simulink library "BPN_lib"  (Simulink 7.4)
settings: Solver=ode45  StartTime=0.0  StopTime=10.0  RelTol=1e-3
values from neighbouring files (symbols this model uses):
  BPNc_fac_ChaPowCurLim = mpt.Parameter    [BPN_CAL.m]
  BPNc_fac_DchPowCurLim = mpt.Parameter    [BPN_CAL.m]
  BPNc_i2_ContiChaCurLim_Max = mpt.Parameter    [BPN_CAL.m]
  BPNc_i2_ContiDchCurLim_Max = mpt.Parameter    [BPN_CAL.m]
  BPNc_i_ContiChaCurLim_Max = mpt.Parameter    [BPN_CAL.m]
  BPNc_i_ContiDchCurLim_Max = mpt.Parameter    [BPN_CAL.m]
  BPNc_i_NorChaCurLim_Max = mpt.Parameter    [BPN_CAL.m]
  BPNc_i_NorDchCurLim_Max = mpt.Parameter    [BPN_CAL.m]
  BPNc_i_PackCurMeasAlwd = mpt.Parameter    [BPN_CAL.m]
  BPNc_i_SafeChaCurLim_Max = mpt.Parameter    [BPN_CAL.m]
  BPNc_i_SafeDchCurLim_Max = mpt.Parameter    [BPN_CAL.m]
  BPNc_pct_CurLimFac_warn = mpt.Parameter    [BPN_CAL.m]
  BPNc_pct_PackSocOver_fatal = mpt.Parameter    [BPN_CAL.m]
  BPNc_pct_PackSocOver_fault = mpt.Parameter    [BPN_CAL.m]
  BPNc_pct_PackSocOver_warn = mpt.Parameter    [BPN_CAL.m]
  BPNc_pct_PackSocUnder_fatal = mpt.Parameter    [BPN_CAL.m]
  BPNc_pct_PackSocUnder_fault = mpt.Parameter    [BPN_CAL.m]
  BPNc_pct_PackSocUnder_warn = mpt.Parameter    [BPN_CAL.m]
  BPNc_pct_PowLimfac_fatal = mpt.Parameter    [BPN_CAL.m]
  BPNc_pct_PowLimfac_warn = mpt.Parameter    [BPN_CAL.m]
  BPNc_r_CtrRes_fault = mpt.Parameter    [BPN_CAL.m]
  BPNc_r_PackInResThrld = mpt.Parameter    [BPN_CAL.m]
  BPNc_t_PackTemp_Mean = mpt.Parameter    [BPN_CAL.m]
  BPNc_v_CellVoltDif_fault = mpt.Parameter    [BPN_CAL.m]
  BPNc_v_CellVoltDif_warn = mpt.Parameter    [BPN_CAL.m]
  BPNc_v_CellVoltOver_fatal = mpt.Parameter    [BPN_CAL.m]
  BPNc_v_CellVoltOver_fault = mpt.Parameter    [BPN_CAL.m]
  BPNc_v_CellVoltOver_warn = mpt.Parameter    [BPN_CAL.m]
  BPNc_v_CellVoltUnder_fatal = mpt.Parameter    [BPN_CAL.m]
  BPNc_v_CellVoltUnder_fault = mpt.Parameter    [BPN_CAL.m]
  BPNc_v_CellVoltUnder_warn = mpt.Parameter    [BPN_CAL.m]
  BPNc_v_LowOPerVolt = mpt.Parameter    [BPN_CAL.m]
  BPNc_v_PackVoltDrop_fatal = mpt.Parameter    [BPN_CAL.m]
  BPNc_v_PackVoltOver_fatal = mpt.Parameter    [BPN_CAL.m]
  BPNc_v_PackVoltOver_fault = mpt.Parameter    [BPN_CAL.m]
  BPNc_v_PackVoltOver_warn = mpt.Parameter    [BPN_CAL.m]
  BPNc_v_PackVoltUnder_fatal = mpt.Parameter    [BPN_CAL.m]
  BPNc_v_PackVoltUnder_fault = mpt.Parameter    [BPN_CAL.m]
  BPNc_v_PackVoltUnder_warn = mpt.Parameter    [BPN_CAL.m]
  BPNc_v_VoltDifThrld = mpt.Parameter    [BPN_CAL.m]
  BPNy_DiagAcvnCtlCtrSt = mpt.Parameter    [BPN_CAL.m]
  BPNz_DiagAcvnCtlId = mpt.Parameter    [BPN_CAL.m]
  BSCx_BCU_State = mpt.Parameter    [BPN_CAL.m]
undefined symbols (not defined in the file or in its folder): BMS_Const_TickTm_s, BPNm_mode_DiaCtlAcv, PACK_Const_CellNumOfMdl, PACK_Const_MdlNumOfPack
libraries: Defined_Functionality x12, simulink x4
(part 1 of 2)
settings Model: Creator=lixuying  LastModifiedBy=sunsijun

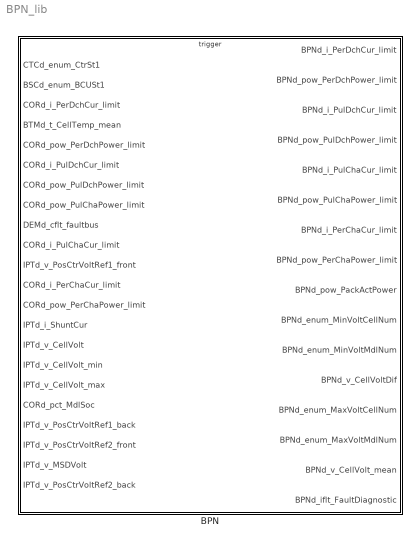
== system BPN_lib ==
  BPN : Subsystem  TreatAsAtomicUnit=on

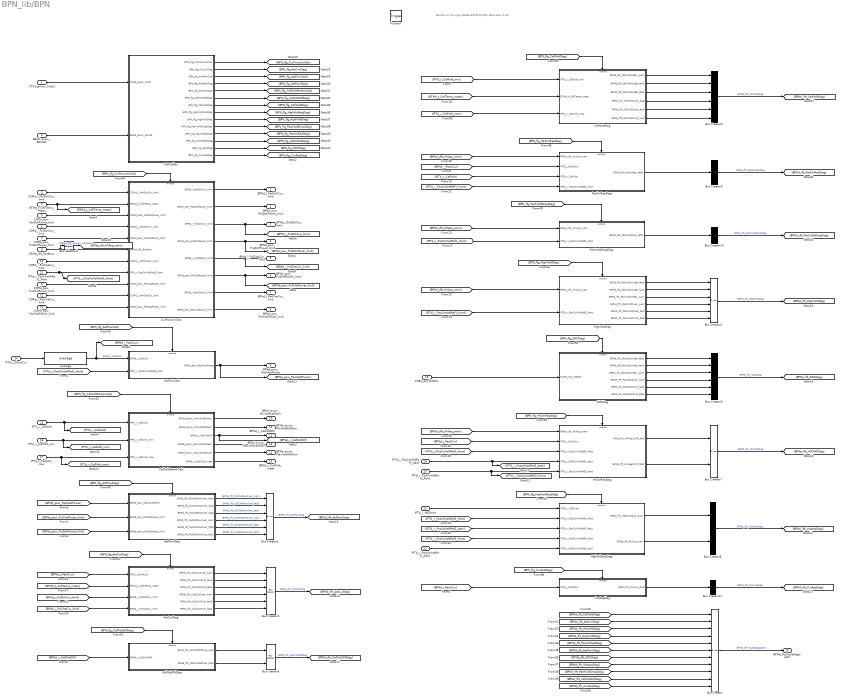
== system BPN_lib/BPN ==
  note: $Author:Li Xuying$
      | $Date:2015/11/03$
      | $Revision:1.0$
  CTCd_enum_CtrSt1 : Inport
  BSCd_enum_BCUSt1 : Inport  Port=2
  CORd_i_PerDchCur_limit : Inport  Port=3
  BTMd_t_CellTemp_mean : Inport  Port=4
  CORd_pow_PerDchPower_limit : Inport  Port=5
  CORd_i_PulDchCur_limit : Inport  Port=6
  CORd_pow_PulDchPower_limit : Inport  Port=7
  CORd_pow_PulChaPower_limit : Inport  Port=8
  DEMd_cflt_faultbus : Inport  Port=9
  CORd_i_PulChaCur_limit : Inport  Port=10
  IPTd_v_PosCtrVoltRef1_front : Inport  Port=11
  CORd_i_PerChaCur_limit : Inport  Port=12
  CORd_pow_PerChaPower_limit : Inport  Port=13
  IPTd_i_ShuntCur : Inport  Port=14
  IPTd_v_CellVolt : Inport  Port=15
  IPTd_v_CellVolt_min : Inport  Port=16
  IPTd_v_CellVolt_max : Inport  Port=17
  CORd_pct_MdlSoc : Inport  Port=18
  IPTd_v_PosCtrVoltRef1_back : Inport  Port=19
  IPTd_v_PosCtrVoltRef2_front : Inport  Port=20
  IPTd_v_MSDVolt : Inport  Port=21
  IPTd_v_PosCtrVoltRef2_back : Inport  Port=22
  function : TriggerPort  TriggerType=function-call
  ActCurDiag : Subsystem
  ActPowCalc : Subsystem
  ActPowDiag : Subsystem
  Bus Creator : BusCreator  Inputs=11
  Bus Creator{1..5} (5 alike) : BusCreator  Inputs=6
  Bus Creator10 : BusCreator  Inputs=1
  Bus Creator11 : BusCreator  Inputs=1
  Bus Creator6 : BusCreator  Inputs=2
  Bus Creator7 : BusCreator  Inputs=2
  Bus Creator8 : BusCreator  Inputs=2
  Bus Creator9 : BusCreator  Inputs=1
  Bus Selector3 : BusSelector  OutputSignals=BPN_Fault_Bus.BPNd_cflt_HVAcq_warnRaw
  CellVoltDiag : Subsystem
  CellVoltDifDiag : Subsystem
  CellVoltParamCalc : Subsystem
  CurAcqDiag : Subsystem
  CurPowLimCalc : Subsystem
  DiaCtrlAcv : Subsystem  TreatAsAtomicUnit=on
  HVCtrResDiag : Subsystem
  HighVoltAcqDiag : Subsystem
  HighVoltDiag : Subsystem
  PackInResDiag : Subsystem
  PackVoltDropDiag : Subsystem
  SOCDiag : Subsystem
  average : Defined_Functionality/average  SystemSampleTime=-1  time=50  period=10
      settings: AttributesFormatString=[TIME_ms=%<time>]\n[PERIOD_ms=%<period>]
  BPNd_i_PerDchCur_limit : Outport
  BPNd_pow_PerDchPower_limit : Outport  Port=2
  BPNd_i_PulDchCur_limit : Outport  Port=3
  BPNd_pow_PulDchPower_limit : Outport  Port=4
  BPNd_i_PulChaCur_limit : Outport  Port=5
  BPNd_pow_PulChaPower_limit : Outport  Port=6
  BPNd_i_PerChaCur_limit : Outport  Port=7
  BPNd_pow_PerChaPower_limit : Outport  Port=8
  BPNd_pow_PackActPower : Outport  Port=9
  BPNd_enum_MinVoltCellNum : Outport  Port=10
  BPNd_enum_MinVoltMdlNum : Outport  Port=11
  BPNd_v_CellVoltDif : Outport  Port=12
  BPNd_enum_MaxVoltCellNum : Outport  Port=13
  BPNd_enum_MaxVoltMdlNum : Outport  Port=14
  BPNd_v_CellVolt_mean : Outport  Port=15
  BPNd_iflt_FaultDiagnostic : Outport  Port=16
  wires:
  CellVoltDiag/6(BPNd_iflt_CellVoltOver_warn) -> Bus Creator3/6
  CellVoltDiag/4(BPNd_iflt_CellVoltOver_fatal) -> Bus Creator3/4
  CurPowLimCalc/6(BPNd_pow_PulChaPower_limit) -> [BPNd_pow_PulChaPower_limit], BPNd_pow_PulChaPower_limit/1
  CurPowLimCalc/5(BPNd_i_PulChaCur_limit) -> [BPNd_i_PulChaCur_limit], BPNd_i_PulChaCur_limit/1
  CurPowLimCalc/4(BPNd_pow_PulDchPower_limit) -> [BPNd_pow_PulDchPower_limit], BPNd_pow_PulDchPower_limit/1
  CurPowLimCalc/3(BPNd_i_PulDchCur_limit) -> [BPNd_i_PulDchCur_limit], BPNd_i_PulDchCur_limit/1
  CurPowLimCalc/2(BPNd_pow_PerDchPower_limit) -> BPNd_pow_PerDchPower_limit/1
  CurPowLimCalc/1(BPNd_i_PerDchCur_limit) -> BPNd_i_PerDchCur_limit/1
  [BPN_flg_HVCtrResDiag] -> HVCtrResDiag/Enable
  [BPN_flg_HighVoltAcqDiag] -> HighVoltAcqDiag/Enable
  DiaCtrlAcv/14(BPN_flg_CurAcqDiag) -> [BPN_flg_CurAcqDiag]
  DiaCtrlAcv/13(BPN_flg_SOCDiag) -> [BPN_flg_SOCDiag]
  DiaCtrlAcv/12(BPN_flg_HVCtrResDiag) -> [BPN_flg_HVCtrResDiag]
  DiaCtrlAcv/11(BPN_flg_PackInResDiag) -> [BPN_flg_PackInResDiag]
  DiaCtrlAcv/10(BPN_flg_PackVoltDropDiag) -> [BPN_flg_PackVoltDropDiag]
  DiaCtrlAcv/9(BPN_flg_HighVoltDiag) -> [BPN_flg_HighVoltDiag]
  DiaCtrlAcv/8(BPN_flg_HighVoltAcqDiag) -> [BPN_flg_HighVoltAcqDiag]
  DiaCtrlAcv/7(BPN_flg_CellVoltDiag) -> [BPN_flg_CellVoltDiag]
  DiaCtrlAcv/6(BPN_flg_CellVoltDifDiag) -> [BPN_flg_CellVoltDifDiag]
  DiaCtrlAcv/5(BPN_flg_CellVoltCalc) -> [BPN_flg_CellVoltParamCalc]
  DiaCtrlAcv/4(BPN_flg_ActPowDiag) -> [BPN_flg_ActPowDiag]
  DiaCtrlAcv/3(BPN_flg_ActPowCalc) -> [BPN_flg_ActPowCalc]
  DiaCtrlAcv/2(BPN_flg_ActCurDiag) -> [BPN_flg_ActCurDiag]
  DiaCtrlAcv/1(BPN_flg_CurPowLimCalc) -> [BPN_flg_CurPowLimCalc]
  Bus Selector3/1 -> [BPNd_cflt_HVAcq_warn]  "<BPNd_cflt_HVAcq_warnRaw>"
  [IPTd_v_PosCtrVoltRef1_back] -> HighVoltAcqDiag/3(IPTd_v_PosCtrVoltRef1_back)
  [IPTd_v_PosCtrVoltRef1_front] -> HighVoltAcqDiag/2(IPTd_v_PosCtrVoltRef1_front)
  IPTd_v_PosCtrVoltRef2_back/1 -> HighVoltAcqDiag/5(IPTd_v_PosCtrVoltRef2_back)
  [IPTd_v_PosCtrVoltRef2_front] -> HighVoltAcqDiag/4(IPTd_v_PosCtrVoltRef2_front)
  HighVoltAcqDiag/1(BPNd_iflt_MSDVoltAcq_warn) -> Bus Creator8/1
  HighVoltAcqDiag/2(BPNd_iflt_HVAcq_warn) -> Bus Creator8/2
  [BPN_flg_CellVoltParamCalc] -> CellVoltParamCalc/Enable
  [BPN_flg_SOCDiag] -> SOCDiag/Enable
  CTCd_enum_CtrSt1/1 -> DiaCtrlAcv/1(CTCd_enum_CtrSt)
  BSCd_enum_BCUSt1/1 -> DiaCtrlAcv/2(BSCd_enum_BCUSt)
  ActPowCalc/1(BPNd_pow_PackActPower) -> [BPNd_pow_PackActPower], BPNd_pow_PackActPower/1
  SOCDiag/6(BPNd_iflt_PackSocOver_fatal) -> Bus Creator5/6
  SOCDiag/5(BPNd_iflt_PackSocOver_fault) -> Bus Creator5/5
  SOCDiag/4(BPNd_iflt_PackSocOver_warn) -> Bus Creator5/4
  SOCDiag/3(BPNd_iflt_PackSocUnder_warn) -> Bus Creator5/3
  SOCDiag/2(BPNd_iflt_PackSocUnder_fault) -> Bus Creator5/2
  SOCDiag/1(BPNd_iflt_PackSocUnder_fatal) -> Bus Creator5/1
  HighVoltDiag/6(BPNd_iflt_PackVoltOver_fatal) -> Bus Creator4/6
  HighVoltDiag/5(BPNd_iflt_PackVoltOver_fault) -> Bus Creator4/5
  HighVoltDiag/4(BPNd_iflt_PackVoltOver_warn) -> Bus Creator4/4
  HighVoltDiag/3(BPNd_iflt_PackVoltUnder_warn) -> Bus Creator4/3
  HighVoltDiag/2(BPNd_iflt_PackVoltUnder_fault) -> Bus Creator4/2
  HighVoltDiag/1(BPNd_iflt_PackVoltUnder_fatal) -> Bus Creator4/1
  CellVoltParamCalc/3(BPNd_v_CellVoltDif) -> [BPNd_v_CellVoltDif], BPNd_v_CellVoltDif/1
  BTMd_t_CellTemp_mean/1 -> [BTMd_t_CellTemp_mean], CurPowLimCalc/2(BTMd_t_CellTemp_mean)
  CORd_pow_PulDchPower_limit/1 -> CurPowLimCalc/5(CORd_pow_PulDchPower_limit)
  CORd_pow_PerDchPower_limit/1 -> CurPowLimCalc/3(CORd_pow_PerDchPower_limit)
  CORd_i_PulChaCur_limit/1 -> CurPowLimCalc/7(CORd_i_PulChaCur_limit)
  CORd_i_PerChaCur_limit/1 -> CurPowLimCalc/10(CORd_i_PerChaCur_limit)
  CORd_pow_PerChaPower_limit/1 -> CurPowLimCalc/11(CORd_pow_PerChaPower_limit)
  CORd_pow_PulChaPower_limit/1 -> CurPowLimCalc/9(CORd_pow_PulChaPower_limit)
  CORd_i_PulDchCur_limit/1 -> CurPowLimCalc/4(CORd_i_PulDchCur_limit)
  CORd_i_PerDchCur_limit/1 -> CurPowLimCalc/1(CORd_i_PerDchCur_limit)
  IPTd_v_PosCtrVoltRef2_front/1 -> [IPTd_v_PosCtrVoltRef2_front], HVCtrResDiag/5(IPTd_v_PosCtrVoltRef2_front)
  IPTd_v_PosCtrVoltRef1_back/1 -> [IPTd_v_PosCtrVoltRef1_back], HVCtrResDiag/4(IPTd_v_PosCtrVoltRef1_back)
  [BPNd_i_PackCur] -> CurAcqDiag/1(IPTd_i_ShuntCur)
  average/1 -> [BPNd_i_PackCur], ActPowCalc/1(BPNd_i_PackCur)  "BPNd_i_PackCur"
  IPTd_v_CellVolt_max/1 -> [IPTd_v_CellVolt_max], CellVoltParamCalc/3(IPTd_v_CellVolt_max)
  [IPTd_v_CellVolt_max] -> CellVoltDiag/3(IPTd_v_CellVolt_max)
  [IPTd_v_CellVolt_min] -> CellVoltDiag/1(IPTd_v_CellVolt_min)
  IPTd_v_CellVolt_min/1 -> [IPTd_v_CellVolt_min], CellVoltParamCalc/2(IPTd_v_CellVolt_min)
  [BPNd_iflt_CurAcqDiag] -> Bus Creator/11
  Bus Creator11/1 -> [BPNd_iflt_CurAcqDiag]  "BPNd_iflt_CurAcqDiag"
  [BPN_flg_CurAcqDiag] -> CurAcqDiag/Enable
  CurAcqDiag/1(BPNd_iflt_CurAcq_fault) -> Bus Creator11/1
  HVCtrResDiag/2(BPNd_iflt_HVNegCtrlR_fault) -> Bus Creator7/2
  HVCtrResDiag/1(BPNd_iflt_HVPosCtrlR_fault) -> Bus Creator7/1
  IPTd_v_MSDVolt/1 -> HighVoltAcqDiag/1(IPTd_v_MSDVolt)
  [BPNd_cflt_HVAcq_warn] -> PackVoltDropDiag/1(BPNd_cflt_HVAcq_warn)
  [IPTd_v_PosCtrVoltRef1_front] -> PackVoltDropDiag/2(IPTd_v_PosCtrVoltRef1_front)
  [IPTd_v_PosCtrVoltRef1_front] -> HighVoltDiag/2(IPTd_v_PosCtrVoltRef1_front)
  DEMd_cflt_faultbus/1 -> Bus Selector3/1, CurPowLimCalc/6(DEMd_cflt_faultbus)
  CurPowLimCalc/8(BPNd_pow_PerChaPower_limit) -> BPNd_pow_PerChaPower_limit/1
  IPTd_i_ShuntCur/1 -> average/1
  [IPTd_v_PosCtrVoltRef1_front] -> ActPowCalc/2(IPTd_v_PosCtrVoltRef1_front)
  [BPNd_pow_PulChaPower_limit] -> ActPowDiag/2(BPNd_pow_PulChaPower_limit)
  [BPNd_pow_PulDchPower_limit] -> ActPowDiag/3(BPNd_pow_PulDchPower_limit)
  [BPNd_pow_PackActPower] -> ActPowDiag/1(BPNd_pow_PackActPower)
  CORd_pct_MdlSoc/1 -> SOCDiag/1(CORd_pct_MdlSoc)
  CellVoltParamCalc/6(BPNd_v_CellVolt_mean) -> BPNd_v_CellVolt_mean/1
  CellVoltParamCalc/1(BPNd_enum_MinVoltCellNum) -> BPNd_enum_MinVoltCellNum/1
  CellVoltParamCalc/2(BPNd_enum_MinVoltMdlNum) -> BPNd_enum_MinVoltMdlNum/1
  CellVoltParamCalc/4(BPNd_enum_MaxVoltCellNum) -> BPNd_enum_MaxVoltCellNum/1
  CellVoltParamCalc/5(BPNd_enum_MaxVoltMdlNum) -> BPNd_enum_MaxVoltMdlNum/1
  [BPNd_v_CellVoltDif] -> CellVoltDifDiag/1(BPNd_v_CellVoltDif)
  CellVoltDifDiag/1(BPNd_iflt_CellVoltDifOver_warn) -> Bus Creator6/1
  CellVoltDifDiag/2(BPNd_iflt_CellVoltDifOver_fault) -> Bus Creator6/2
  [BPNd_i_PackCur] -> ActCurDiag/1(IPTd_i_ShuntCur)
  IPTd_v_CellVolt/1 -> [IPTd_v_CellVolt], CellVoltParamCalc/1(IPTd_v_CellVolt)
  PackInResDiag/1(BPNd_iflt_PackInRes_fatal) -> Bus Creator9/1
  [BPNd_i_PackCur] -> PackInResDiag/2(IPTd_i_ShuntCur)
  [IPTd_v_CellVolt] -> PackInResDiag/3(IPTd_v_CellVolt)
  IPTd_v_PosCtrVoltRef1_front/1 -> CurPowLimCalc/8(IPTd_v_PosCtrVoltRef1_front), [IPTd_v_PosCtrVoltRef1_front]
  [IPTd_v_PosCtrVoltRef1_front] -> PackInResDiag/4(IPTd_v_PosCtrVoltRef1_front)
  [BPNd_i_PackCur] -> HVCtrResDiag/2(IPTd_i_ShuntCur)
  [IPTd_v_PosCtrVoltRef1_front] -> HVCtrResDiag/3(IPTd_v_PosCtrVoltRef1_front)
  [BTMd_t_CellTemp_mean] -> ActCurDiag/2(BTMd_t_CellTemp_mean)
  [BTMd_t_CellTemp_mean] -> CellVoltDiag/2(BTMd_t_CellTemp_mean)
  [BPNd_i_PulDchCur_limit] -> ActCurDiag/3(BPNd_i_PulDchCur_limit)
  [BPNd_i_PulChaCur_limit] -> ActCurDiag/4(BPNd_i_PulChaCur_limit)
  CurPowLimCalc/7(BPNd_i_PerChaCur_limit) -> BPNd_i_PerChaCur_limit/1
  ActPowDiag/1(BPNd_iflt_PulChaPowOver_warn) -> Bus Creator1/1  "BPNd_iflt_PulChaPowOver_warn"
  ActPowDiag/2(BPNd_iflt_PulChaPowOver_fault) -> Bus Creator1/2  "BPNd_iflt_PulChaPowOver_fault"
  ActPowDiag/3(BPNd_iflt_PulChaPowOver_fatal) -> Bus Creator1/3  "BPNd_iflt_PulChaPowOver_fatal"
  ActPowDiag/4(BPNd_iflt_PulDchPowOver_warn) -> Bus Creator1/4  "BPNd_iflt_PulDchPowOver_warn"
  ActPowDiag/5(BPNd_iflt_PulDchPowOver_fatal) -> Bus Creator1/5  "BPNd_iflt_PulDchPowOver_fatal"
  ActPowDiag/6(BPNd_iflt_PulDchPowOver_fault) -> Bus Creator1/6  "BPNd_iflt_PulDchPowOver_fault"
  [BPNd_cflt_HVAcq_warn] -> HVCtrResDiag/1(BPNd_cflt_HVAcq_warn)
  PackVoltDropDiag/1(BPNd_ilft_PackVoltDrop_fatal) -> Bus Creator10/1
  [BPNd_cflt_HVAcq_warn] -> PackInResDiag/1(BPNd_cflt_HVAcq_warn)
  [BPNd_cflt_HVAcq_warn] -> HighVoltDiag/1(BPNd_cflt_HVAcq_warn)
  Bus Creator/1 -> BPNd_iflt_FaultDiagnostic/1  "BPNd_iflt_FaultDiagnostic"
  Bus Creator1/1 -> [BPNd_iflt_ActPowDiag]  "BPNd_iflt_ActPowDiag"
  ActCurDiag/1(BPNd_iflt_DchCurOver_warn) -> Bus Creator2/1
  ActCurDiag/2(BPNd_iflt_DchCurOver_fault) -> Bus Creator2/2
  ActCurDiag/3(BPNd_iflt_DchCurOver_fatal) -> Bus Creator2/3
  ActCurDiag/4(BPNd_iflt_ChaCurOver_warn) -> Bus Creator2/4
  ActCurDiag/5(BPNd_iflt_ChaCurOver_fault) -> Bus Creator2/5
  ActCurDiag/6(BPNd_iflt_ChaCurOver_fatal) -> Bus Creator2/6
  Bus Creator2/1 -> [BPNd_iflt_ActCurDiag]  "BPNd_iflt_ActCurDiag"
  Bus Creator3/1 -> [BPNd_iflt_CellVoltDiag]  "BPNd_iflt_CellVoltDiag"
  CellVoltDiag/1(BPNd_iflt_CellVoltUnder_warn) -> Bus Creator3/1
  CellVoltDiag/2(BPNd_iflt_CellVoltUnder_fault) -> Bus Creator3/2
  CellVoltDiag/3(BPNd_iflt_CellVoltUnder_fatal) -> Bus Creator3/3
  CellVoltDiag/5(BPNd_iflt_CellVoltOver_fault) -> Bus Creator3/5
  Bus Creator4/1 -> [BPNd_iflt_HighVoltDiag]  "BPNd_iflt_HighVoltDiag"
  Bus Creator5/1 -> [BPNd_iflt_SOCDiag]  "BPNd_iflt_SOCDiag"
  Bus Creator7/1 -> [BPNd_iflt_HVCtrRDiag]  "BPNd_iflt_HVCtrRDiag"
  [BPNd_iflt_CellVoltDiag] -> Bus Creator/1
  [BPNd_iflt_ActCurDiag] -> Bus Creator/2
  [BPNd_iflt_HVCtrRDiag] -> Bus Creator/3
  [BPNd_iflt_HighVoltDiag] -> Bus Creator/4
  [BPNd_iflt_PackInResDiag] -> Bus Creator/5
  [BPNd_iflt_ActPowDiag] -> Bus Creator/6
  [BPNd_iflt_SOCDiag] -> Bus Creator/7
  [BPNd_iflt_VoltAcqDiag] -> Bus Creator/8
  [BPNd_ilft_PackVoltDropDiag] -> Bus Creator/9
  Bus Creator6/1 -> [BPNd_iflt_CellVoltDifDiag]  "BPNd_iflt_CellVoltDifDiag"
  Bus Creator8/1 -> [BPNd_iflt_VoltAcqDiag]  "BPNd_iflt_VoltAcqDiag"
  Bus Creator9/1 -> [BPNd_iflt_PackInResDiag]  "BPNd_iflt_PackInResDiag"
  Bus Creator10/1 -> [BPNd_ilft_PackVoltDropDiag]  "BPNd_ilft_PackVoltDropDiag"
  [BPNd_iflt_CellVoltDifDiag] -> Bus Creator/10
  [BPN_flg_CurPowLimCalc] -> CurPowLimCalc/Enable
  [BPN_flg_ActPowCalc] -> ActPowCalc/Enable
  [BPN_flg_ActPowDiag] -> ActPowDiag/Enable
  [BPN_flg_ActCurDiag] -> ActCurDiag/Enable
  [BPN_flg_PackInResDiag] -> PackInResDiag/Enable
  [BPN_flg_PackVoltDropDiag] -> PackVoltDropDiag/Enable
  [BPN_flg_CellVoltDiag] -> CellVoltDiag/Enable
  [BPN_flg_CellVoltDifDiag] -> CellVoltDifDiag/Enable
  [BPN_flg_HighVoltDiag] -> HighVoltDiag/Enable

== system BPN_lib/BPN/ActCurDiag ==
  IPTd_i_ShuntCur : Inport
  BTMd_t_CellTemp_mean : Inport  Port=2
  BPNd_i_PulDchCur_limit : Inport  Port=3
  BPNd_i_PulChaCur_limit : Inport  Port=4
  Enable : EnablePort
  ChaCurDiag : Subsystem  TreatAsAtomicUnit=on
  DchCurDiag : Subsystem  TreatAsAtomicUnit=on
  If : If
  Subsystem : Subsystem
  BPNd_iflt_DchCurOver_warn : Outport
  BPNd_iflt_DchCurOver_fault : Outport  Port=2
  BPNd_iflt_DchCurOver_fatal : Outport  Port=3
  BPNd_iflt_ChaCurOver_warn : Outport  Port=4
  BPNd_iflt_ChaCurOver_fault : Outport  Port=5
  BPNd_iflt_ChaCurOver_fatal : Outport  Port=6
  wires:
  [BPN_i_PulChaCur_LimitAbs] -> ChaCurDiag/3(BPNd_i_PulChaCur_limit)
  [BTMd_t_CellTemp_mean] -> ChaCurDiag/1(BTMd_t_CellTemp_mean)
  Subsystem/1(BPN_i_PulDchCur_limit) -> DchCurDiag/2(BPNd_i_PulDchCur_limit)
  BTMd_t_CellTemp_mean/1 -> [BTMd_t_CellTemp_mean], DchCurDiag/3(BTMd_t_CellTemp_mean)
  BPNd_i_PulChaCur_limit/1 -> Subsystem/2(BPNd_i_PulChaCur_limit)
  Subsystem/2(BPN_i_PulChaCur_LimitAbs) -> [BPN_i_PulChaCur_LimitAbs]
  BPNd_i_PulDchCur_limit/1 -> Subsystem/1(BPNd_i_PulDchCur_limit)
  ChaCurDiag/1(BPNd_iflt_ChaCurOver_fault) -> BPNd_iflt_ChaCurOver_fault/1
  ChaCurDiag/2(BPNd_iflt_ChaCurOver_warn) -> BPNd_iflt_ChaCurOver_warn/1
  [IPTd_i_ShuntCur] -> ChaCurDiag/2(IPTd_i_ShuntCur)
  [IPTd_i_ShuntCur] -> DchCurDiag/1(IPTd_i_PackCur)
  IPTd_i_ShuntCur/1 -> [IPTd_i_ShuntCur], If/1
  ChaCurDiag/3(BPNd_iflt_ChaCurOver_fatal) -> BPNd_iflt_ChaCurOver_fatal/1
  DchCurDiag/3(BPNd_iflt_DchCurOver_fatal) -> BPNd_iflt_DchCurOver_fatal/1
  DchCurDiag/1(BPNd_iflt_DchCurOver_warn) -> BPNd_iflt_DchCurOver_warn/1
  DchCurDiag/2(BPNd_iflt_DchCurOver_fault) -> BPNd_iflt_DchCurOver_fault/1
  If/2 -> ChaCurDiag/Action
  If/1 -> DchCurDiag/Action

== system BPN_lib/BPN/ActPowCalc ==
  BPNd_i_PackCur : Inport
  IPTd_v_PosCtrVoltRef1_front : Inport  Port=2
  Enable : EnablePort
  Product : Product  RndMeth=Zero
  BPNd_pow_PackActPower : Outport
  wires:
  IPTd_v_PosCtrVoltRef1_front/1 -> Product/2
  Product/1 -> BPNd_pow_PackActPower/1  "BPNd_pow_PackActPower"
  BPNd_i_PackCur/1 -> Product/1

== system BPN_lib/BPN/ActPowDiag ==
  BPNd_pow_PackActPower : Inport
  BPNd_pow_PulChaPower_limit : Inport  Port=2
  BPNd_pow_PulDchPower_limit : Inport  Port=3
  Enable : EnablePort
  If : If  IfExpression=u1 < 0
  PulChaPower_Diagnosic : Subsystem  TreatAsAtomicUnit=on
  PulDchPower_Diagnosic : Subsystem  TreatAsAtomicUnit=on
  BPNd_iflt_PulChaPowOver_warn : Outport  DataType=boolean  OutDataTypeStr=boolean
  BPNd_iflt_PulChaPowOver_fault : Outport  Port=2  DataType=boolean  OutDataTypeStr=boolean
  BPNd_iflt_PulChaPowOver_fatal : Outport  Port=3  DataType=boolean  OutDataTypeStr=boolean
  BPNd_iflt_PulDchPowOver_warn : Outport  Port=4  DataType=boolean  OutDataTypeStr=boolean
  BPNd_iflt_PulDchPowOver_fatal : Outport  Port=5  DataType=boolean  OutDataTypeStr=boolean
  BPNd_iflt_PulDchPowOver_fault : Outport  Port=6  DataType=boolean  OutDataTypeStr=boolean  InitialOutput=0
  wires:
  [BPNd_pow_PackActPower] -> PulDchPower_Diagnosic/2(BPNd_pow_PackActPower)
  [BPNd_pow_PackActPower] -> PulChaPower_Diagnosic/1(BPNd_pow_PackActPower)
  BPNd_pow_PulChaPower_limit/1 -> PulChaPower_Diagnosic/2(BPNd_pow_PulChaPower_limit)
  PulChaPower_Diagnosic/3(BPNd_iflt_PulChaPowOver_fatal) -> BPNd_iflt_PulChaPowOver_fatal/1
  PulChaPower_Diagnosic/2(BPNd_iflt_PulChaPowOver_fault) -> BPNd_iflt_PulChaPowOver_fault/1
  PulChaPower_Diagnosic/1(BPNd_iflt_PulChaPowOver_warn) -> BPNd_iflt_PulChaPowOver_warn/1
  PulDchPower_Diagnosic/2(BPNd_iflt_PulDchPowOver_fault) -> BPNd_iflt_PulDchPowOver_fault/1
  BPNd_pow_PackActPower/1 -> [BPNd_pow_PackActPower], If/1
  PulDchPower_Diagnosic/1(BPNd_iflt_PulDchPowOver_warn) -> BPNd_iflt_PulDchPowOver_warn/1
  PulDchPower_Diagnosic/3(BPNd_iflt_PulDchPowOver_fatal) -> BPNd_iflt_PulDchPowOver_fatal/1
  BPNd_pow_PulDchPower_limit/1 -> PulDchPower_Diagnosic/1(BPNd_pow_PulDchPower_limit)
  If/1 -> PulChaPower_Diagnosic/Action
  If/2 -> PulDchPower_Diagnosic/Action

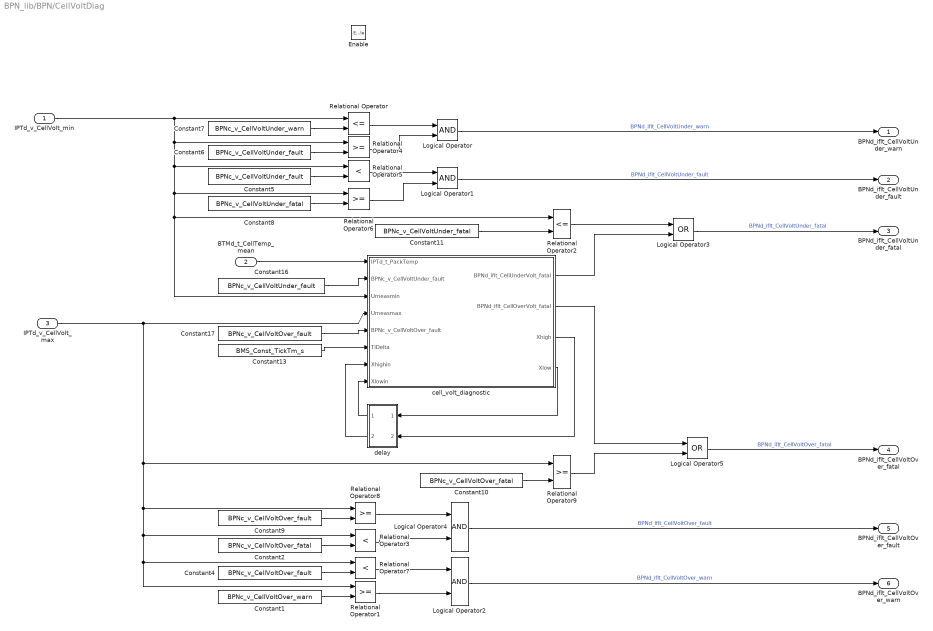
== system BPN_lib/BPN/CellVoltDiag ==
  IPTd_v_CellVolt_min : Inport
  BTMd_t_CellTemp_mean : Inport  Port=2
  IPTd_v_CellVolt_max : Inport  Port=3
  Enable : EnablePort
  Constant1 : Constant  Value=BPNc_v_CellVoltOver_warn
  Constant10 : Constant  Value=BPNc_v_CellVoltOver_fatal
  Constant11 : Constant  Value=BPNc_v_CellVoltUnder_fatal
  Constant13 : Constant  Value=BMS_Const_TickTm_s  OutDataTypeMode=single  OutDataTypeStr=single
  Constant16 : Constant  Value=BPNc_v_CellVoltUnder_fault  OutDataTypeMode=single  OutDataTypeStr=single
  Constant17 : Constant  Value=BPNc_v_CellVoltOver_fault  OutDataTypeMode=single  OutDataTypeStr=single
  Constant2 : Constant  Value=BPNc_v_CellVoltOver_fatal
  Constant4 : Constant  Value=BPNc_v_CellVoltOver_fault
  Constant5 : Constant  Value=BPNc_v_CellVoltUnder_fault
  Constant6 : Constant  Value=BPNc_v_CellVoltUnder_fault
  Constant7 : Constant  Value=BPNc_v_CellVoltUnder_warn
  Constant8 : Constant  Value=BPNc_v_CellVoltUnder_fatal
  Constant9 : Constant  Value=BPNc_v_CellVoltOver_fault
  Logical Operator{,1..2,4} (4 alike) : Logic  AllPortsSameDT=off  OutDataTypeMode=boolean  OutDataTypeStr=boolean
  Logical Operator3 : Logic  Operator=OR  AllPortsSameDT=off  OutDataTypeMode=boolean  OutDataTypeStr=boolean
  Logical Operator5 : Logic  Operator=OR  AllPortsSameDT=off  OutDataTypeMode=boolean  OutDataTypeStr=boolean
  Relational Operator : RelationalOperator  Operator=<=  LogicOutDataTypeMode=boolean  OutDataTypeStr=boolean
  Relational Operator{1,4,6,8..9} (5 alike) : RelationalOperator  LogicOutDataTypeMode=boolean  OutDataTypeStr=boolean
  Relational Operator2 : RelationalOperator  Operator=<=  LogicOutDataTypeMode=boolean  OutDataTypeStr=boolean
  Relational Operator3 : RelationalOperator  Operator=<  LogicOutDataTypeMode=boolean  OutDataTypeStr=boolean
  Relational Operator5 : RelationalOperator  Operator=<  LogicOutDataTypeMode=boolean  OutDataTypeStr=boolean
  Relational Operator7 : RelationalOperator  Operator=<  LogicOutDataTypeMode=boolean  OutDataTypeStr=boolean
  cell_volt_diagnostic : Stateflow chart  TreatAsAtomicUnit=on
  delay : Subsystem
  BPNd_iflt_CellVoltUnder_warn : Outport
  BPNd_iflt_CellVoltUnder_fault : Outport  Port=2
  BPNd_iflt_CellVoltUnder_fatal : Outport  Port=3
  BPNd_iflt_CellVoltOver_fatal : Outport  Port=4
  BPNd_iflt_CellVoltOver_fault : Outport  Port=5
  BPNd_iflt_CellVoltOver_warn : Outport  Port=6
  wires:
  IPTd_v_CellVolt_min/1 -> Relational Operator2/1, cell_volt_diagnostic/3(Umeasmin), Relational Operator6/1, Relational Operator5/1, Relational Operator4/1, Relational Operator/1
  Logical Operator5/1 -> BPNd_iflt_CellVoltOver_fatal/1  "BPNd_iflt_CellVoltOver_fatal"
  Relational Operator9/1 -> Logical Operator5/2
  cell_volt_diagnostic/2(BPNd_iflt_CellOverVolt_fatal) -> Logical Operator5/1
  Constant10/1 -> Relational Operator9/2
  Logical Operator4/1 -> BPNd_iflt_CellVoltOver_fault/1  "BPNd_iflt_CellVoltOver_fault"
  Relational Operator3/1 -> Logical Operator4/2
  Relational Operator8/1 -> Logical Operator4/1
  Constant9/1 -> Relational Operator8/2
  Logical Operator2/1 -> BPNd_iflt_CellVoltOver_warn/1  "BPNd_iflt_CellVoltOver_warn"
  Relational Operator1/1 -> Logical Operator2/2
  Relational Operator7/1 -> Logical Operator2/1
  Constant4/1 -> Relational Operator7/2
  Logical Operator3/1 -> BPNd_iflt_CellVoltUnder_fatal/1  "BPNd_iflt_CellVoltUnder_fatal"
  cell_volt_diagnostic/1(BPNd_iflt_CellUnderVolt_fatal) -> Logical Operator3/2
  Relational Operator2/1 -> Logical Operator3/1
  Logical Operator1/1 -> BPNd_iflt_CellVoltUnder_fault/1  "BPNd_iflt_CellVoltUnder_fault"
  Constant8/1 -> Relational Operator6/2
  Relational Operator6/1 -> Logical Operator1/2
  Relational Operator5/1 -> Logical Operator1/1
  Constant5/1 -> Relational Operator5/2
  Logical Operator/1 -> BPNd_iflt_CellVoltUnder_warn/1  "BPNd_iflt_CellVoltUnder_warn"
  Relational Operator4/1 -> Logical Operator/2
  Relational Operator/1 -> Logical Operator/1
  Constant6/1 -> Relational Operator4/2
  Constant7/1 -> Relational Operator/2
  BTMd_t_CellTemp_mean/1 -> cell_volt_diagnostic/1(IPTd_t_PackTemp)
  Constant17/1 -> cell_volt_diagnostic/5(BPNc_v_CellVoltOver_fault)
  Constant16/1 -> cell_volt_diagnostic/2(BPNc_v_CellVoltUnder_fault)
  Constant13/1 -> cell_volt_diagnostic/6(TiDelta)
  Constant2/1 -> Relational Operator3/2
  Constant11/1 -> Relational Operator2/2
  Constant1/1 -> Relational Operator1/2
  IPTd_v_CellVolt_max/1 -> Relational Operator9/1, Relational Operator8/1, Relational Operator7/1, Relational Operator1/1, Relational Operator3/1, cell_volt_diagnostic/4(Umeasmax)
  delay/2(Out2) -> cell_volt_diagnostic/7(Xhighin)
  delay/1(Out1) -> cell_volt_diagnostic/8(Xlowin)
  cell_volt_diagnostic/4(Xlow) -> delay/1(In1)
  cell_volt_diagnostic/3(Xhigh) -> delay/2(In2)

== system BPN_lib/BPN/CellVoltDifDiag ==
  BPNd_v_CellVoltDif : Inport
  Enable : EnablePort
  Constant : Constant  Value=BPNc_v_CellVoltDif_warn  OutDataTypeMode=single  OutDataTypeStr=single
  Constant1 : Constant  Value=BPNc_v_CellVoltDif_fault  OutDataTypeMode=single  OutDataTypeStr=single
  Logical Operator : Logic  AllPortsSameDT=off  OutDataTypeMode=boolean  OutDataTypeStr=boolean
  Relational Operator : RelationalOperator  LogicOutDataTypeMode=boolean  OutDataTypeStr=boolean
  Relational Operator1 : RelationalOperator  Operator=<=  LogicOutDataTypeMode=boolean  OutDataTypeStr=boolean
  Relational Operator2 : RelationalOperator  Operator=<  LogicOutDataTypeMode=boolean  OutDataTypeStr=boolean
  BPNd_iflt_CellVoltDifOver_warn : Outport
  BPNd_iflt_CellVoltDifOver_fault : Outport  Port=2
  wires:
  Logical Operator/1 -> BPNd_iflt_CellVoltDifOver_warn/1  "BPNd_iflt_CellVoltDifOver_warn"
  Relational Operator2/1 -> Logical Operator/2
  Relational Operator/1 -> Logical Operator/1
  Relational Operator1/1 -> BPNd_iflt_CellVoltDifOver_fault/1  "BPNd_iflt_CellVoltDifOver_fault"
  Constant1/1 -> Relational Operator1/1, Relational Operator2/2
  Constant/1 -> Relational Operator/2
  BPNd_v_CellVoltDif/1 -> Relational Operator1/2, Relational Operator2/1, Relational Operator/1

== system BPN_lib/BPN/CellVoltParamCalc ==
  IPTd_v_CellVolt : Inport
  IPTd_v_CellVolt_min : Inport  Port=2
  IPTd_v_CellVolt_max : Inport  Port=3
  Enable : EnablePort
  Constant1 : Constant  Value=PACK_Const_MdlNumOfPack  OutDataTypeMode=uint8  OutDataTypeStr=uint8
  Constant2 : Constant  Value=PACK_Const_CellNumOfMdl  OutDataTypeMode=uint8  OutDataTypeStr=uint8
  Constant3 : Constant  Value=PACK_Const_MdlNumOfPack  OutDataTypeMode=uint8  OutDataTypeStr=uint8
  Constant4 : Constant  Value=PACK_Const_CellNumOfMdl  OutDataTypeMode=uint8  OutDataTypeStr=uint8
  Divide : Product  Inputs=*/
  MaxVoltLocationCalc : Stateflow chart  TreatAsAtomicUnit=on
  MinVoltLocationCalc : Stateflow chart  TreatAsAtomicUnit=on
  Reshape : Reshape  OutputDimensionality=Customize  OutputDimensions=[5,32]
  Subtract : Sum  Inputs=-+
  Sum of Elements : Sum  Inputs=+
  Width : Width  DataType=single
  BPNd_enum_MinVoltCellNum : Outport
  BPNd_enum_MinVoltMdlNum : Outport  Port=2
  BPNd_v_CellVoltDif : Outport  Port=3
  BPNd_enum_MaxVoltCellNum : Outport  Port=4
  BPNd_enum_MaxVoltMdlNum : Outport  Port=5
  BPNd_v_CellVolt_mean : Outport  Port=6
  wires:
  Constant2/1 -> MinVoltLocationCalc/1(PACK_Const_CellNumOfMdl)
  Subtract/1 -> BPNd_v_CellVoltDif/1  "BPNd_v_CellVoltDif"
  Constant4/1 -> MaxVoltLocationCalc/2(PACK_Const_CellNumOfMdl)
  Constant1/1 -> MinVoltLocationCalc/2(PACK_Const_MdlNumOfPack)
  MaxVoltLocationCalc/1(BPNd_enum_MaxVoltCellNum) -> BPNd_enum_MaxVoltCellNum/1
  [BPNd_v_CellVoltReshap] -> MaxVoltLocationCalc/4(BPNd_v_CellVoltReshap)
  Reshape/1 -> MinVoltLocationCalc/3(BPNd_v_CellVoltReshap), [BPNd_v_CellVoltReshap]
  Constant3/1 -> MaxVoltLocationCalc/3(PACK_Const_MdlNumOfPack)
  MaxVoltLocationCalc/2(BPNd_enum_MaxVoltMdlNum) -> BPNd_enum_MaxVoltMdlNum/1
  MinVoltLocationCalc/1(BPNd_enum_MinVoltCellNum) -> BPNd_enum_MinVoltCellNum/1
  MinVoltLocationCalc/2(BPNd_enum_MinVoltMdlNum) -> BPNd_enum_MinVoltMdlNum/1
  IPTd_v_CellVolt/1 -> Sum of Elements/1, Width/1, Reshape/1
  Width/1 -> Divide/2
  Divide/1 -> BPNd_v_CellVolt_mean/1  "BPNd_v_CellVolt_mean"
  Sum of Elements/1 -> Divide/1
  IPTd_v_CellVolt_max/1 -> MaxVoltLocationCalc/1(BPNd_v_CellMaxVolt), Subtract/2
  IPTd_v_CellVolt_min/1 -> MinVoltLocationCalc/4(BPNd_v_CellMinVolt), Subtract/1

== system BPN_lib/BPN/CurAcqDiag ==
  IPTd_i_ShuntCur : Inport
  Enable : EnablePort
  Ground : Ground
  Terminator : Terminator
  BPNd_iflt_CurAcq_fault : Outport  OutDataType=fixdt(1, 16)  OutScaling=2^0
  wires:
  IPTd_i_ShuntCur/1 -> Terminator/1
  Ground/1 -> BPNd_iflt_CurAcq_fault/1  "BPNd_iflt_CurAcq_fault"

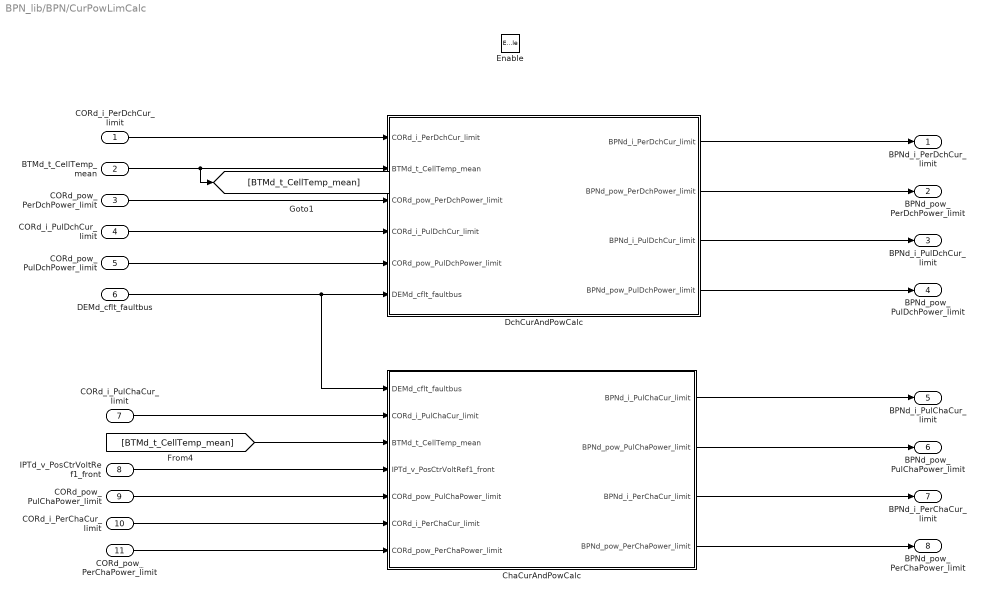
== system BPN_lib/BPN/CurPowLimCalc ==
  CORd_i_PerDchCur_limit : Inport
  BTMd_t_CellTemp_mean : Inport  Port=2
  CORd_pow_PerDchPower_limit : Inport  Port=3
  CORd_i_PulDchCur_limit : Inport  Port=4  DataType=single  OutDataTypeStr=single
  CORd_pow_PulDchPower_limit : Inport  Port=5
  DEMd_cflt_faultbus : Inport  Port=6
  CORd_i_PulChaCur_limit : Inport  Port=7
  IPTd_v_PosCtrVoltRef1_front : Inport  Port=8
  CORd_pow_PulChaPower_limit : Inport  Port=9
  CORd_i_PerChaCur_limit : Inport  Port=10
  CORd_pow_PerChaPower_limit : Inport  Port=11
  Enable : EnablePort
  ChaCurAndPowCalc : Subsystem  TreatAsAtomicUnit=on
  DchCurAndPowCalc : Subsystem  TreatAsAtomicUnit=on
  BPNd_i_PerDchCur_limit : Outport  DataType=single  OutDataTypeStr=single
  BPNd_pow_PerDchPower_limit : Outport  Port=2  DataType=single  OutDataTypeStr=single
  BPNd_i_PulDchCur_limit : Outport  Port=3
  BPNd_pow_PulDchPower_limit : Outport  Port=4
  BPNd_i_PulChaCur_limit : Outport  Port=5
  BPNd_pow_PulChaPower_limit : Outport  Port=6
  BPNd_i_PerChaCur_limit : Outport  Port=7
  BPNd_pow_PerChaPower_limit : Outport  Port=8
  wires:
  DchCurAndPowCalc/4(BPNd_pow_PulDchPower_limit) -> BPNd_pow_PulDchPower_limit/1
  DchCurAndPowCalc/3(BPNd_i_PulDchCur_limit) -> BPNd_i_PulDchCur_limit/1
  DchCurAndPowCalc/2(BPNd_pow_PerDchPower_limit) -> BPNd_pow_PerDchPower_limit/1
  DchCurAndPowCalc/1(BPNd_i_PerDchCur_limit) -> BPNd_i_PerDchCur_limit/1
  [BTMd_t_CellTemp_mean] -> ChaCurAndPowCalc/3(BTMd_t_CellTemp_mean)
  CORd_pow_PerChaPower_limit/1 -> ChaCurAndPowCalc/7(CORd_pow_PerChaPower_limit)
  CORd_i_PerChaCur_limit/1 -> ChaCurAndPowCalc/6(CORd_i_PerChaCur_limit)
  CORd_pow_PulChaPower_limit/1 -> ChaCurAndPowCalc/5(CORd_pow_PulChaPower_limit)
  IPTd_v_PosCtrVoltRef1_front/1 -> ChaCurAndPowCalc/4(IPTd_v_PosCtrVoltRef1_front)
  CORd_i_PulChaCur_limit/1 -> ChaCurAndPowCalc/2(CORd_i_PulChaCur_limit)
  CORd_pow_PulDchPower_limit/1 -> DchCurAndPowCalc/5(CORd_pow_PulDchPower_limit)
  CORd_i_PulDchCur_limit/1 -> DchCurAndPowCalc/4(CORd_i_PulDchCur_limit)
  CORd_pow_PerDchPower_limit/1 -> DchCurAndPowCalc/3(CORd_pow_PerDchPower_limit)
  BTMd_t_CellTemp_mean/1 -> [BTMd_t_CellTemp_mean], DchCurAndPowCalc/2(BTMd_t_CellTemp_mean)
  CORd_i_PerDchCur_limit/1 -> DchCurAndPowCalc/1(CORd_i_PerDchCur_limit)
  ChaCurAndPowCalc/4(BPNd_pow_PerChaPower_limit) -> BPNd_pow_PerChaPower_limit/1
  ChaCurAndPowCalc/3(BPNd_i_PerChaCur_limit) -> BPNd_i_PerChaCur_limit/1
  ChaCurAndPowCalc/2(BPNd_pow_PulChaPower_limit) -> BPNd_pow_PulChaPower_limit/1
  ChaCurAndPowCalc/1(BPNd_i_PulChaCur_limit) -> BPNd_i_PulChaCur_limit/1
  DEMd_cflt_faultbus/1 -> ChaCurAndPowCalc/1(DEMd_cflt_faultbus), DchCurAndPowCalc/6(DEMd_cflt_faultbus)

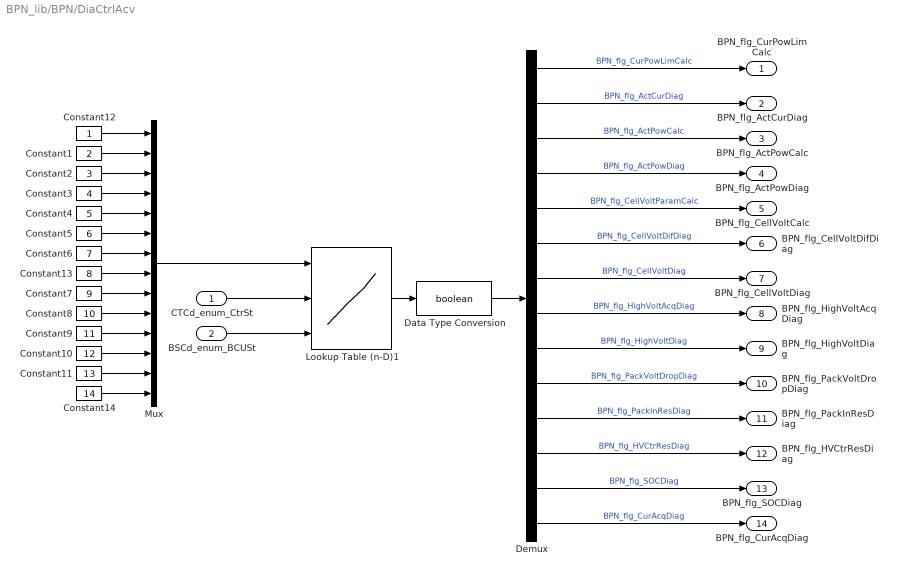
== system BPN_lib/BPN/DiaCtrlAcv ==
  CTCd_enum_CtrSt : Inport
  BSCd_enum_BCUSt : Inport  Port=2
  Constant1 : Constant  Value=2  OutDataTypeMode=uint8  OutDataTypeStr=uint8
  Constant10 : Constant  Value=12  OutDataTypeMode=uint8  OutDataTypeStr=uint8
  Constant11 : Constant  Value=13  OutDataTypeMode=uint8  OutDataTypeStr=uint8
  Constant12 : Constant  OutDataTypeMode=uint8  OutDataTypeStr=uint8
  Constant13 : Constant  Value=8  OutDataTypeMode=uint8  OutDataTypeStr=uint8
  Constant14 : Constant  Value=14  OutDataTypeMode=uint8  OutDataTypeStr=uint8
  Constant2 : Constant  Value=3  OutDataTypeMode=uint8  OutDataTypeStr=uint8
  Constant3 : Constant  Value=4  OutDataTypeMode=uint8  OutDataTypeStr=uint8
  Constant4 : Constant  Value=5  OutDataTypeMode=uint8  OutDataTypeStr=uint8
  Constant5 : Constant  Value=6  OutDataTypeMode=uint8  OutDataTypeStr=uint8
  Constant6 : Constant  Value=7  OutDataTypeMode=uint8  OutDataTypeStr=uint8
  Constant7 : Constant  Value=9  OutDataTypeMode=uint8  OutDataTypeStr=uint8
  Constant8 : Constant  Value=10  OutDataTypeMode=uint8  OutDataTypeStr=uint8
  Constant9 : Constant  Value=11  OutDataTypeMode=uint8  OutDataTypeStr=uint8
  Data Type Conversion : DataTypeConversion  OutDataTypeMode=boolean  OutDataTypeStr=boolean
  Demux : Demux  Outputs=14
  Lookup Table (n-D)1 : Lookup_n-D  NumberOfTableDimensions=3  BreakpointsForDimension1=BPNz_DiagAcvnCtlId  BreakpointsForDimension2=BPNy_DiagAcvnCtlCtrSt  BreakpointsForDimension3=BSCx_BCU_State  BreakpointsForDimension1DataTypeStr=uint8  BreakpointsForDimension2DataTypeStr=uint8  BreakpointsForDimension3DataTypeStr=uint8  Table=BPNm_mode_DiaCtlAcv  IntermediateResultsDataTypeStr=uint8  InterpMethod=None - Flat  OutDataTypeStr=uint8  RndMeth=Nearest  FractionDataTypeStr=single  InputSameDT=on
  Mux : Mux  Inputs=14
  BPN_flg_CurPowLimCalc : Outport  DataType=boolean  OutDataTypeStr=boolean
  BPN_flg_ActCurDiag : Outport  Port=2  DataType=boolean  OutDataTypeStr=boolean
  BPN_flg_ActPowCalc : Outport  Port=3  DataType=boolean  OutDataTypeStr=boolean
  BPN_flg_ActPowDiag : Outport  Port=4  DataType=boolean  OutDataTypeStr=boolean
  BPN_flg_CellVoltCalc : Outport  Port=5  DataType=boolean  OutDataTypeStr=boolean
  BPN_flg_CellVoltDifDiag : Outport  Port=6  DataType=boolean  OutDataTypeStr=boolean
  BPN_flg_CellVoltDiag : Outport  Port=7  DataType=boolean  OutDataTypeStr=boolean
  BPN_flg_HighVoltAcqDiag : Outport  Port=8  DataType=boolean  OutDataTypeStr=boolean
  BPN_flg_HighVoltDiag : Outport  Port=9  DataType=boolean  OutDataTypeStr=boolean
  BPN_flg_PackVoltDropDiag : Outport  Port=10  DataType=boolean  OutDataTypeStr=boolean
  BPN_flg_PackInResDiag : Outport  Port=11  DataType=boolean  OutDataTypeStr=boolean
  BPN_flg_HVCtrResDiag : Outport  Port=12  DataType=boolean  OutDataTypeStr=boolean
  BPN_flg_SOCDiag : Outport  Port=13  DataType=boolean  OutDataTypeStr=boolean
  BPN_flg_CurAcqDiag : Outport  Port=14  DataType=boolean  OutDataTypeStr=boolean
  wires:
  Demux/8 -> BPN_flg_HighVoltAcqDiag/1  "BPN_flg_HighVoltAcqDiag"
  Demux/14 -> BPN_flg_CurAcqDiag/1  "BPN_flg_CurAcqDiag"
  Constant14/1 -> Mux/14
  Constant11/1 -> Mux/13
  Constant10/1 -> Mux/12
  Constant9/1 -> Mux/11
  Constant8/1 -> Mux/10
  Constant7/1 -> Mux/9
  Constant13/1 -> Mux/8
  Constant12/1 -> Mux/1
  Constant1/1 -> Mux/2
  Constant2/1 -> Mux/3
  Constant3/1 -> Mux/4
  Constant4/1 -> Mux/5
  Constant5/1 -> Mux/6
  Constant6/1 -> Mux/7
  Data Type Conversion/1 -> Demux/1
  Demux/7 -> BPN_flg_CellVoltDiag/1  "BPN_flg_CellVoltDiag"
  Demux/9 -> BPN_flg_HighVoltDiag/1  "BPN_flg_HighVoltDiag"
  Demux/11 -> BPN_flg_PackInResDiag/1  "BPN_flg_PackInResDiag"
  Demux/12 -> BPN_flg_HVCtrResDiag/1  "BPN_flg_HVCtrResDiag"
  Demux/13 -> BPN_flg_SOCDiag/1  "BPN_flg_SOCDiag"
  Demux/1 -> BPN_flg_CurPowLimCalc/1  "BPN_flg_CurPowLimCalc"
  Demux/2 -> BPN_flg_ActCurDiag/1  "BPN_flg_ActCurDiag"
  Demux/3 -> BPN_flg_ActPowCalc/1  "BPN_flg_ActPowCalc"
  Demux/4 -> BPN_flg_ActPowDiag/1  "BPN_flg_ActPowDiag"
  Demux/5 -> BPN_flg_CellVoltCalc/1  "BPN_flg_CellVoltParamCalc"
  Demux/6 -> BPN_flg_CellVoltDifDiag/1  "BPN_flg_CellVoltDifDiag"
  Demux/10 -> BPN_flg_PackVoltDropDiag/1  "BPN_flg_PackVoltDropDiag"
  Lookup Table (n-D)1/1 -> Data Type Conversion/1
  BSCd_enum_BCUSt/1 -> Lookup Table (n-D)1/3
  CTCd_enum_CtrSt/1 -> Lookup Table (n-D)1/2
  Mux/1 -> Lookup Table (n-D)1/1

== system BPN_lib/BPN/HVCtrResDiag ==
  BPNd_cflt_HVAcq_warn : Inport
  IPTd_i_ShuntCur : Inport  Port=2
  IPTd_v_PosCtrVoltRef1_front : Inport  Port=3
  IPTd_v_PosCtrVoltRef1_back : Inport  Port=4
  IPTd_v_PosCtrVoltRef2_front : Inport  Port=5
  Enable : EnablePort  StatesWhenEnabling=reset
  Compare To Constant : simulink/Logic and Bit Operations/Compare To Constant  SystemSampleTime=-1  relop=~=  const=1  LogicOutDataTypeMode=uint8
  Constant1 : Constant  Value=BPNc_i_PackCurMeasAlwd
  HVCtrResDiag : Subsystem
  Logical Operator : Logic  AllPortsSameDT=off  OutDataTypeMode=boolean  OutDataTypeStr=boolean
  Relational Operator1 : RelationalOperator  LogicOutDataTypeMode=boolean  OutDataTypeStr=boolean
  BPNd_iflt_HVPosCtrlR_fault : Outport
  BPNd_iflt_HVNegCtrlR_fault : Outport  Port=2
  wires:
  [IPTd_i_DCLinkCur] -> HVCtrResDiag/3(IPTd_i_DCLinkCur)
  IPTd_v_PosCtrVoltRef2_front/1 -> HVCtrResDiag/4(IPTd_v_PosCtrVoltRef2_front)
  Logical Operator/1 -> HVCtrResDiag/Enable
  Relational Operator1/1 -> Logical Operator/2
  Compare To Constant/1 -> Logical Operator/1
  BPNd_cflt_HVAcq_warn/1 -> Compare To Constant/1
  IPTd_v_PosCtrVoltRef1_back/1 -> HVCtrResDiag/2(IPTd_v_PosCtrVoltRef1_back)
  IPTd_v_PosCtrVoltRef1_front/1 -> HVCtrResDiag/1(IPTd_v_PosCtrVoltRef1_front)
  HVCtrResDiag/2(BPNd_iflt_HVNegCtrlR_fault) -> BPNd_iflt_HVNegCtrlR_fault/1
  HVCtrResDiag/1(BPNd_iflt_HVPosCtrlR_fault) -> BPNd_iflt_HVPosCtrlR_fault/1
  Constant1/1 -> Relational Operator1/2
  IPTd_i_ShuntCur/1 -> [IPTd_i_DCLinkCur], Relational Operator1/1

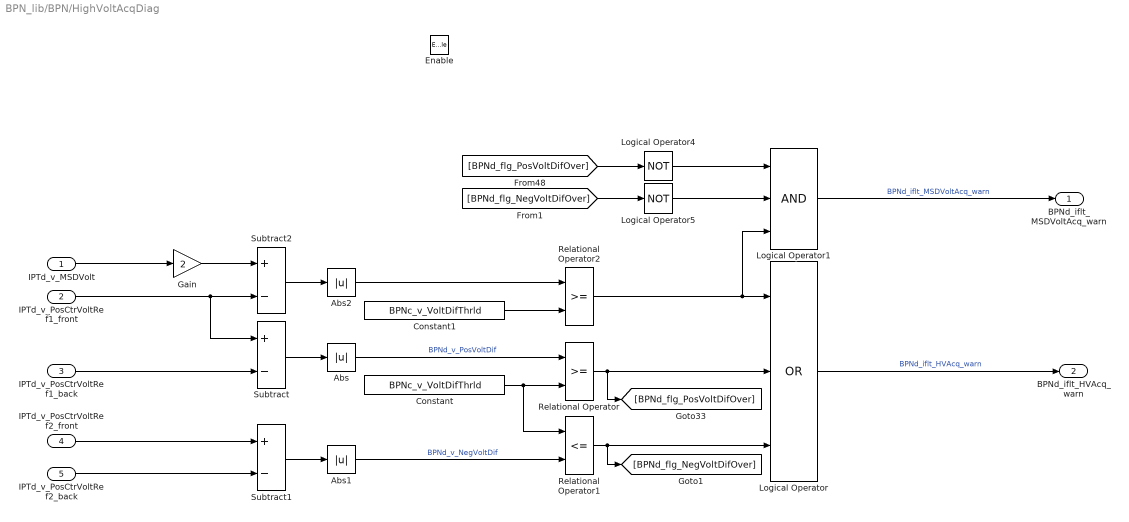
== system BPN_lib/BPN/HighVoltAcqDiag ==
  IPTd_v_MSDVolt : Inport
  IPTd_v_PosCtrVoltRef1_front : Inport  Port=2
  IPTd_v_PosCtrVoltRef1_back : Inport  Port=3
  IPTd_v_PosCtrVoltRef2_front : Inport  Port=4
  IPTd_v_PosCtrVoltRef2_back : Inport  Port=5
  Enable : EnablePort
  Abs : Abs
  Abs1 : Abs
  Abs2 : Abs
  Constant : Constant  Value=BPNc_v_VoltDifThrld
  Constant1 : Constant  Value=BPNc_v_VoltDifThrld
  Gain : Gain  Gain=2  ParameterDataType=fixdt(1, 16)  ParameterScaling=2^0  OutDataType=fixdt(1, 16)  OutScaling=2^0
  Logical Operator : Logic  Operator=OR  Inputs=3  AllPortsSameDT=off  OutDataTypeMode=boolean  OutDataTypeStr=boolean
  Logical Operator1 : Logic  Inputs=3  AllPortsSameDT=off  OutDataTypeMode=boolean  LogicDataType=fixdt(0, 8)  OutDataTypeStr=boolean
  Logical Operator4 : Logic  Operator=NOT  AllPortsSameDT=off  OutDataTypeMode=boolean  LogicDataType=fixdt(0, 8)  OutDataTypeStr=boolean
  Logical Operator5 : Logic  Operator=NOT  AllPortsSameDT=off  OutDataTypeMode=boolean  LogicDataType=fixdt(0, 8)  OutDataTypeStr=boolean
  Relational Operator : RelationalOperator  LogicOutDataTypeMode=boolean  OutDataTypeStr=boolean
  Relational Operator1 : RelationalOperator  Operator=<=  LogicOutDataTypeMode=boolean  OutDataTypeStr=boolean
  Relational Operator2 : RelationalOperator  LogicOutDataTypeMode=boolean  OutDataTypeStr=boolean
  Subtract : Sum  Inputs=+-
  Subtract1 : Sum  Inputs=+-
  Subtract2 : Sum  Inputs=+-
  BPNd_iflt_MSDVoltAcq_warn : Outport
  BPNd_iflt_HVAcq_warn : Outport  Port=2
  wires:
  [BPNd_flg_NegVoltDifOver] -> Logical Operator5/1
  [BPNd_flg_PosVoltDifOver] -> Logical Operator4/1
  Logical Operator5/1 -> Logical Operator1/2
  Logical Operator4/1 -> Logical Operator1/1
  Constant/1 -> Relational Operator1/1, Relational Operator/2
  Logical Operator/1 -> BPNd_iflt_HVAcq_warn/1  "BPNd_iflt_HVAcq_warn"
  Logical Operator1/1 -> BPNd_iflt_MSDVoltAcq_warn/1  "BPNd_iflt_MSDVoltAcq_warn"
  Relational Operator/1 -> Logical Operator/2, [BPNd_flg_PosVoltDifOver]
  Relational Operator2/1 -> Logical Operator1/3, Logical Operator/1
  Constant1/1 -> Relational Operator2/2
  Abs2/1 -> Relational Operator2/1
  Subtract2/1 -> Abs2/1
  Gain/1 -> Subtract2/1
  IPTd_v_MSDVolt/1 -> Gain/1
  IPTd_v_PosCtrVoltRef2_back/1 -> Subtract1/2
  IPTd_v_PosCtrVoltRef2_front/1 -> Subtract1/1
  Subtract1/1 -> Abs1/1
  Abs1/1 -> Relational Operator1/2  "BPNd_v_NegVoltDif"
  Relational Operator1/1 -> Logical Operator/3, [BPNd_flg_NegVoltDifOver]
  IPTd_v_PosCtrVoltRef1_front/1 -> Subtract/1, Subtract2/2
  IPTd_v_PosCtrVoltRef1_back/1 -> Subtract/2
  Subtract/1 -> Abs/1
  Abs/1 -> Relational Operator/1  "BPNd_v_PosVoltDif"

== system BPN_lib/BPN/HighVoltDiag ==
  BPNd_cflt_HVAcq_warn : Inport
  IPTd_v_PosCtrVoltRef1_front : Inport  Port=2
  Enable : EnablePort
  Compare To Constant : simulink/Logic and Bit Operations/Compare To Constant  SystemSampleTime=-1  relop=~=  const=1  LogicOutDataTypeMode=uint8
  HighVoltDiag : Subsystem
  BPNd_iflt_PackVoltUnder_fatal : Outport
  BPNd_iflt_PackVoltUnder_fault : Outport  Port=2
  BPNd_iflt_PackVoltUnder_warn : Outport  Port=3
  BPNd_iflt_PackVoltOver_warn : Outport  Port=4
  BPNd_iflt_PackVoltOver_fault : Outport  Port=5
  BPNd_iflt_PackVoltOver_fatal : Outport  Port=6
  wires:
  HighVoltDiag/3(BPNd_iflt_PackVoltUnder_warn) -> BPNd_iflt_PackVoltUnder_warn/1
  HighVoltDiag/2(BPNd_iflt_PackVoltUnder_fault) -> BPNd_iflt_PackVoltUnder_fault/1
  HighVoltDiag/1(BPNd_iflt_PackVoltUnder_fatal) -> BPNd_iflt_PackVoltUnder_fatal/1
  HighVoltDiag/6(BPNd_iflt_PackVoltOver_fatal) -> BPNd_iflt_PackVoltOver_fatal/1
  HighVoltDiag/5(BPNd_iflt_PackVoltOver_fault) -> BPNd_iflt_PackVoltOver_fault/1
  HighVoltDiag/4(BPNd_iflt_PackVoltOver_warn) -> BPNd_iflt_PackVoltOver_warn/1
  Compare To Constant/1 -> HighVoltDiag/Enable
  BPNd_cflt_HVAcq_warn/1 -> Compare To Constant/1
  IPTd_v_PosCtrVoltRef1_front/1 -> HighVoltDiag/1(IPTd_v_PosCtrVoltRef1_front)

== system BPN_lib/BPN/PackInResDiag ==
  BPNd_cflt_HVAcq_warn : Inport
  IPTd_i_ShuntCur : Inport  Port=2
  IPTd_v_CellVolt : Inport  Port=3
  IPTd_v_PosCtrVoltRef1_front : Inport  Port=4
  Enable : EnablePort  StatesWhenEnabling=reset
  Abs : Abs  OutDataType=fixdt(1, 16)  OutScaling=2^0
  Compare To Constant : simulink/Logic and Bit Operations/Compare To Constant  SystemSampleTime=-1  relop=~=  const=1  LogicOutDataTypeMode=boolean
  Constant1 : Constant  Value=BPNc_i_PackCurMeasAlwd
  Logical Operator : Logic  AllPortsSameDT=off  OutDataTypeMode=boolean  OutDataTypeStr=boolean
  PackInResDiag : Subsystem
  Relational Operator1 : RelationalOperator  LogicOutDataTypeMode=boolean  OutDataTypeStr=boolean
  BPNd_iflt_PackInRes_fatal : Outport
  wires:
  [BPNd_i_DClinkCurAbs] -> PackInResDiag/3(BPNd_i_DClinkCurAbs)
  Abs/1 -> [BPNd_i_DClinkCurAbs], Relational Operator1/1
  Logical Operator/1 -> PackInResDiag/Enable
  Relational Operator1/1 -> Logical Operator/2
  Compare To Constant/1 -> Logical Operator/1
  BPNd_cflt_HVAcq_warn/1 -> Compare To Constant/1
  IPTd_v_PosCtrVoltRef1_front/1 -> PackInResDiag/2(IPTd_v_PosCtrVoltRef1_front)
  PackInResDiag/1(BPNd_iflt_PackInRes_fatal) -> BPNd_iflt_PackInRes_fatal/1
  IPTd_v_CellVolt/1 -> PackInResDiag/1(IPTd_v_CellVolt)
  Constant1/1 -> Relational Operator1/2
  IPTd_i_ShuntCur/1 -> Abs/1

== system BPN_lib/BPN/PackVoltDropDiag ==
  BPNd_cflt_HVAcq_warn : Inport
  IPTd_v_PosCtrVoltRef1_front : Inport  Port=2
  Enable : EnablePort
  Compare To Constant : simulink/Logic and Bit Operations/Compare To Constant  SystemSampleTime=-1  relop=~=  const=1  LogicOutDataTypeMode=uint8
  PackVoltDropDiag : Subsystem
  BPNd_ilft_PackVoltDrop_fatal : Outport
  wires:
  IPTd_v_PosCtrVoltRef1_front/1 -> PackVoltDropDiag/1(IPTd_v_PosCtrVoltRef1_front)
  BPNd_cflt_HVAcq_warn/1 -> Compare To Constant/1
  PackVoltDropDiag/1(BPNd_ilft_PackVoltDrop_fatal) -> BPNd_ilft_PackVoltDrop_fatal/1
  Compare To Constant/1 -> PackVoltDropDiag/Enable

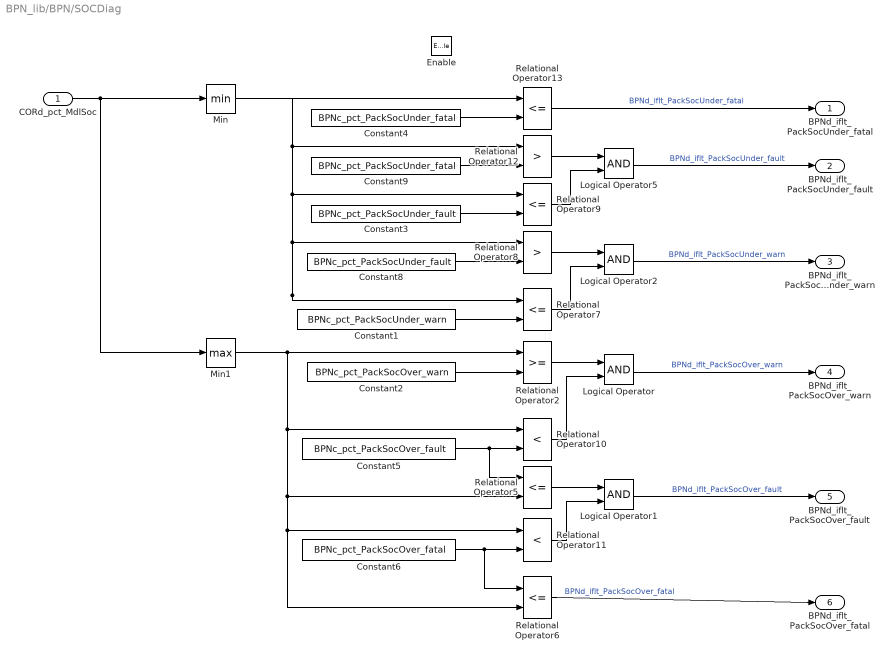
== system BPN_lib/BPN/SOCDiag ==
  CORd_pct_MdlSoc : Inport
  Enable : EnablePort
  Constant1 : Constant  Value=BPNc_pct_PackSocUnder_warn  OutDataTypeMode=single  OutDataTypeStr=single
  Constant2 : Constant  Value=BPNc_pct_PackSocOver_warn  OutDataTypeMode=single  OutDataTypeStr=single
  Constant3 : Constant  Value=BPNc_pct_PackSocUnder_fault  OutDataTypeMode=single  OutDataTypeStr=single
  Constant4 : Constant  Value=BPNc_pct_PackSocUnder_fatal  OutDataTypeMode=single  OutDataTypeStr=single
  Constant5 : Constant  Value=BPNc_pct_PackSocOver_fault  OutDataTypeMode=single  OutDataTypeStr=single
  Constant6 : Constant  Value=BPNc_pct_PackSocOver_fatal  OutDataTypeMode=single  OutDataTypeStr=single
  Constant8 : Constant  Value=BPNc_pct_PackSocUnder_fault  OutDataTypeMode=single  OutDataTypeStr=single
  Constant9 : Constant  Value=BPNc_pct_PackSocUnder_fatal  OutDataTypeMode=single  OutDataTypeStr=single
  Logical Operator{,1..2,5} (4 alike) : Logic  AllPortsSameDT=off  OutDataTypeMode=boolean  OutDataTypeStr=boolean
  Min : MinMax
  Min1 : MinMax  Function=max
  Relational Operator10 : RelationalOperator  Operator=<  LogicOutDataTypeMode=boolean  OutDataTypeStr=boolean
  Relational Operator11 : RelationalOperator  Operator=<  LogicOutDataTypeMode=boolean  OutDataTypeStr=boolean
  Relational Operator12 : RelationalOperator  Operator=>  LogicOutDataTypeMode=boolean  OutDataTypeStr=boolean
  Relational Operator{5..7,9,13} (5 alike) : RelationalOperator  Operator=<=  LogicOutDataTypeMode=boolean  OutDataTypeStr=boolean
  Relational Operator2 : RelationalOperator  LogicOutDataTypeMode=boolean  OutDataTypeStr=boolean
  Relational Operator8 : RelationalOperator  Operator=>  LogicOutDataTypeMode=boolean  OutDataTypeStr=boolean
  BPNd_iflt_PackSocUnder_fatal : Outport
  BPNd_iflt_PackSocUnder_fault : Outport  Port=2
  BPNd_iflt_PackSocUnder_warn : Outport  Port=3
  BPNd_iflt_PackSocOver_warn : Outport  Port=4
  BPNd_iflt_PackSocOver_fault : Outport  Port=5
  BPNd_iflt_PackSocOver_fatal : Outport  Port=6
  wires:
  Constant6/1 -> Relational Operator6/1, Relational Operator11/2
  Constant5/1 -> Relational Operator5/1, Relational Operator10/2
  Min1/1 -> Relational Operator11/1, Relational Operator6/2, Relational Operator5/2, Relational Operator10/1, Relational Operator2/1
  Min/1 -> Relational Operator7/1, Relational Operator8/1, Relational Operator9/1, Relational Operator12/1, Relational Operator13/1
  CORd_pct_MdlSoc/1 -> Min1/1, Min/1
  Constant4/1 -> Relational Operator13/2
  Constant9/1 -> Relational Operator12/2
  Constant3/1 -> Relational Operator9/2
  Constant8/1 -> Relational Operator8/2
  Constant1/1 -> Relational Operator7/2
  Relational Operator13/1 -> BPNd_iflt_PackSocUnder_fatal/1  "BPNd_iflt_PackSocUnder_fatal"
  Logical Operator5/1 -> BPNd_iflt_PackSocUnder_fault/1  "BPNd_iflt_PackSocUnder_fault"
  Logical Operator2/1 -> BPNd_iflt_PackSocUnder_warn/1  "BPNd_iflt_PackSocUnder_warn"
  Constant2/1 -> Relational Operator2/2
  Relational Operator2/1 -> Logical Operator/1
  Relational Operator10/1 -> Logical Operator/2
  Relational Operator5/1 -> Logical Operator1/1
  Relational Operator11/1 -> Logical Operator1/2
  Relational Operator7/1 -> Logical Operator2/2
  Relational Operator8/1 -> Logical Operator2/1
  Relational Operator12/1 -> Logical Operator5/1
  Relational Operator9/1 -> Logical Operator5/2
  Logical Operator1/1 -> BPNd_iflt_PackSocOver_fault/1  "BPNd_iflt_PackSocOver_fault"
  Logical Operator/1 -> BPNd_iflt_PackSocOver_warn/1  "BPNd_iflt_PackSocOver_warn"
  Relational Operator6/1 -> BPNd_iflt_PackSocOver_fatal/1  "BPNd_iflt_PackSocOver_fatal"
